simulink model "Ej3_Perassi"  (R2023b)
settings: Solver=ode4  StartTime=0.0  StopTime=10.0  FixedStep=0.0001  RelTol=1e-3
values from neighbouring files (symbols this model uses):
  ue = x3e    [EJ2_Perassi.m]
  x1e = pi / 6    (= 0.523598775598)    [EJ2_Perassi.m]
  x2e = 0    [EJ2_Perassi.m]
  x3e = a * abs(x1e) * x1e - sin(x1e)    [EJ2_Perassi.m]
  ye = x1e    (= 0.523598775598)    [EJ2_Perassi.m]
libraries: cstblocks x1
settings Model: Creator=aghersin  LastModifiedBy=Usuario
settings DataIOCC: ReturnWorkspaceOutputs=off
settings OptimizationCC: LifeSpan=inf
settings DebuggingCC: UnconnectedInputMsg=warning  UnconnectedOutputMsg=warning  UnconnectedLineMsg=warning  SFExecutionAtInitializationDiag=none  ArithmeticOperatorsInVariantConditions=warning
settings ModelReferenceCC: EnableRefExpFcnMdlSchedulingChecks=on
settings SFSimCC: SimUseLocalCustomCode=off  CustomCodeUndefinedFunction=UseInterfaceOnly
settings RTWCC: RTWUseLocalCustomCode=off
settings CodeAppCC: StateflowObjectComments=on

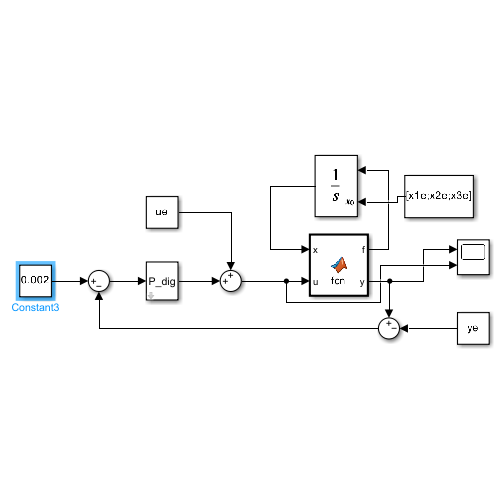
[thumbnail: Simulink's stored preview of the top-level diagram]
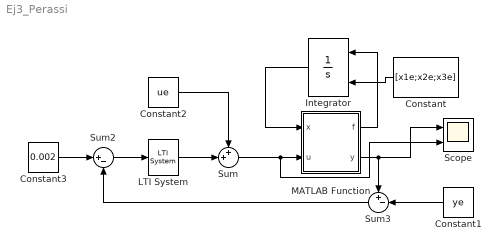
== system Ej3_Perassi ==
  Constant : Constant  Value=[x1e;x2e;x3e]
  Constant1 : Constant  Value=ye
  Constant2 : Constant  Value=ue
  Constant3 : Constant  Value=0.002
  Integrator : Integrator  InitialConditionSource=external
  LTI System : cstblocks/LTI System  sys=P_dig  IC=[]  PadeOrder=0
  MATLAB Function : MATLAB Function  TreatAsAtomicUnit=on
  Scope : Scope  NumInputPorts=2
  Sum : Sum  Inputs=++|
  Sum2 : Sum  Inputs=|+-
  Sum3 : Sum  Inputs=+-|
  wires:
  Integrator/1 -> MATLAB Function/1(x)
  MATLAB Function/1(f) -> Integrator/1
  Constant/1 -> Integrator/2
  MATLAB Function/2(y) -> Sum3/1, Scope/1
  Constant1/1 -> Sum3/2
  Constant2/1 -> Sum/1
  Sum2/1 -> LTI System/1
  Constant3/1 -> Sum2/1
  Sum3/1 -> Sum2/2
  LTI System/1 -> Sum/2
  Sum/1 -> Scope/2, MATLAB Function/2(u)

== matlab function Ej3_Perassi/MATLAB Function ==
  data: x input; u input; f output; y output
function [f,y] = fcn(x,u)

f1 = x(2);
f2 = -0.25 * (6 / pi)^2 * x(1)^2 + sin(x(1)) - x(2)^2 + x(3);
f3 = 20 * u - 20 * x(3);


f=[f1;f2;f3];

y=x(1);
